simulink model "IntModelY1_2022a"  (R2022a)
settings: Solver=VariableStepAuto  StartTime=0.0  StopTime=inf  RelTol=1e-3
model workspace (MAT data in the model file):
  firstWarning = 1
  originalScenarioChecksum = '114339432DE22364D47BB28FC96DC10C'
undefined symbols (not defined in the file): Acceleration, ActorID, AngularVelocity, curvature, curvatureAhd, DefaultGear, DEND_B, DEND_S, DEND_T, direction, driving, gradbp, L, LF, LR, matlabshared, MAX_BRAKE, MAX_STEER, MAX_TORQUE, MCAR, MIN_BRAKE, MIN_STEER, MIN_TORQUE, NUMD_B, NUMD_S, NUMD_T, Pitch, Position, psi_o, R, Roll, RRdamp, SceneInfo, session, sigbuilder_block, STEER_RATIO, stopSign_ID, Tdead, thetaRefs, TL_ID, TrackWidth, Ts, ts, Vdead, Velocity, WB, X_o, xRef2s, Y_o, Yaw, yRef2s
libraries: drivingscenarioandsensors x8, drivingvehiclecontroller x2, trackingutilitieslib x2, simulink x2, robotalgslib x1, mpcadaslib x1, drivinglib x1, simulink_extras x1, autolibshared x1, vehdynlibviscommon x1, vehdynlibsteering x1
(part 3 of 3)

== stateflow chart IntModelY1_2022a/Behavioural Planner/Routing ==
  state InitialRoute
    en:
    NewRoute = 0;
  state Rerouting
    en:
    NewRoute = 1;
  (default) -> InitialRoute
  InitialRoute -> Rerouting : [ReRoute == 1]
  Rerouting -> InitialRoute : [ReRoute == 0]
  data: ReRoute input; NewRoute output

== matlab function IntModelY1_2022a/Environment & Data/Sensors & Perception/MATLAB Function1 ==
  data: EVpos input; yaw input; SceneID input; SceneInfo input; SDir output; SDist input; D2S output
function [SDir,D2S] = SceneFinder(EVpos,yaw, SceneID, SceneInfo, SDist)
D2S = zeros(10,1);
    % dist = zeros(1,length(SceneLocations));
    for j = 1:length(SceneInfo(:,1))
        distXY = SceneInfo(j,1:2) - EVpos(1:2);
        D2S(j) = norm(distXY);
        
%         if (D2S <= SDist)
%             Scene = SceneInfo(j,3); % labels {1,2,3,4} => {'TrafficLight','StopSign','RailRoadCrossing','RoundAbout'};
%             angl = atan2d(distXY(2),distXY(1));
%             angl = angl - yaw;
% %             rot = [cosd(angl) -sind(angl);sind(angl) cosd(angl)];
% %             distXY = rot*distXY';
% %             angl = atan2d(distXY(2),distXY(1));
%             
%             if angl < 0
%                 angl = angl + 360;
%             end
% 
%             if (angl > 315) || (angl <= 45) 
%                 SDir = "N";
%             elseif (angl > 225) && (angl <= 315)
%                 SDir = "E";
%             elseif (angl > 135) && (angl <= 225)
%                 SDir = "S";
%                 D2S = 1000;
%                 angl = 1000;
%                 Scene = 0;
%             elseif (angl > 45) && (angl <= 135)
%                 SDir = "W";
%             else
%                 SDir = "Error";
%             end
%             break
%         else
%             Scene = 0;
%             SDir = " ";
%             angl = 1000;
%             D2S = 1000;
%         end

    end
[val,indx] = min(D2S);

== stateflow chart IntModelY1_2022a/Behavioural Planner/Emergency Stop ==
  state EmergencyCheck
    en:
    EStop = 0;
  state Pullover
    en:
    EStop=1;
  state Stop
    en:
    EStop=2;
  Pullover -> EmergencyCheck : [TechFailure == 0]
  (default) -> EmergencyCheck
  EmergencyCheck -> Pullover [order 1] : [TechFailure == 1]
  EmergencyCheck -> Stop [order 2] : [D2O<=1]
  Stop -> EmergencyCheck : [D2O > 2]
  data: D2O input; TechFailure input; EStop output

== stateflow chart IntModelY1_2022a/Behavioural Planner/Collision Avoidance ==
  state Start
    en:
    Stuck = 0;
    ACC = 0;
    LaneChangeCmd = 0;
    %VelCmd = CurrentVelCmd;
  state Follow
    en:
    ACC = 1;
  state LaneChange
    en:
    LaneChangeCmd = 1;
  LaneChange -> Start : [LaneChanged == 1]
  (default) -> Start
  Follow -> LaneChange [order 2] : [LaneAvailable == 1 && Stuck == 1]
  Start -> Follow : [ObjAhead == 1]
  Follow -> Start [order 3] : [ObjAhead == 0]
  Follow -> Follow [order 1] : [(EgoSpeed <= MinSpeed) && after(WaitTime,sec)]{Stuck = 1;}
  data: Stuck local; ACC output; WaitTime input; ObjAhead input; MinSpeed input; LaneAvailable input; EgoSpeed input; LaneChanged input; LaneChangeCmd output

== matlab function IntModelY1_2022a/Controllers/Subsystem3/Subsystem2/MATLAB Function ==
  data: u input; accel output; decel output
function [accel, decel] = fcn(u)
if(u>0)
    accel=u; decel=0;
elseif(u<0)
    accel=0; decel=-u;
else
    accel=0;decel=0;
end

== matlab function IntModelY1_2022a/Controllers/MATLAB Function2 ==
  data: v input; RefVelCmd output; curvature input
function RefVelCmd = fcn(v,curvature)

    if abs(curvature) >= 0 && abs(curvature) <= 1e-2
        RefVelCmd = v;
    else
        r = 1/abs(curvature);
        RefVelCmd = min(v,sqrt(9.81*r*.7));
    end

== matlab function IntModelY1_2022a/Vehicle Dynamics/Info2ActorState/MATLAB Function1 ==
  data: Xdot input; Velocity output; Ydot input; Zdot input
function Velocity = fcn(Xdot, Ydot, Zdot)

Velocity = [Xdot Ydot, Zdot];

== matlab function IntModelY1_2022a/Behavioural Planner/MATLAB Function ==
  data: Dest input; D2D output; CurrentPose input
function D2D = fcn(Dest, CurrentPose)
CurrentPose(2) = -CurrentPose(2);
D2D = norm(Dest - CurrentPose(1:2)');

== matlab function IntModelY1_2022a/Vehicle Dynamics/Info2ActorState/MATLAB Function2 ==
  data: aX input; Acceleration output; aY input; aZ input
function Acceleration = fcn(aX, aY, aZ)

Acceleration = [aX aY, aZ];

== matlab function IntModelY1_2022a/Vehicle Dynamics/Info2ActorState/MATLAB Function3 ==
  data: phiDot input; AngularVelocity output; thetaDot input; psiDot input
function AngularVelocity = fcn(phiDot, thetaDot, psiDot)

AngularVelocity = [phiDot thetaDot, psiDot];

== stateflow chart IntModelY1_2022a/Vehicle Dynamics/VehicleDynamics/engine-steer-brake dynamics/GearSelection1 ==
  state Park
    CurrGear = 0;
  state Reverse
    CurrGear = -1;
  state drive
    CurrGear = 1;
  (default) -> (junction 12)
  (junction 12) -> Reverse [order 3] : [DefaultGear == -1]
  (junction 12) -> drive [order 2] : [DefaultGear == 1]
  (junction 12) -> Park [order 1] : [DefaultGear == 0]
  (junction 12) -> Park [order 4] : %fallback to park
  drive -> Park [order 2] : [gear_cmd == 0 && allowShift(vc,Tbrake)]
  Park -> Reverse [order 2] : [gear_cmd == -1 && allowShift(vc,Tbrake)]
  Park -> drive [order 1] : [gear_cmd == 1 && allowShift(vc,Tbrake)]
  Reverse -> Park [order 2] : [gear_cmd == 0 && allowShift(vc,Tbrake)]
  drive -> Reverse [order 1] : [gear_cmd == -1 && allowShift(vc,Tbrake)]
  Reverse -> drive [order 1] : [gear_cmd == 1 && allowShift(vc,Tbrake)]
  data: Tdead parameter; Vdead parameter; vel function_input; brakeT function_input; allow function_output; CurrGear output; Tbrake input; vc input; gear_cmd input; DefaultGear parameter
  function allow = allowShift(vel, brakeT):
    | function allow = allowShift(vel, brakeT)
    | allow = (abs(vel) <= Vdead) && (abs(brakeT)>Tdead);
    | end

== matlab function IntModelY1_2022a/Vehicle Dynamics/VehicleDynamics/engine-steer-brake dynamics/compute net torque ==
  data: gear input; Tnet output; Tengine input; Tbrake input; vc input
function Tnet  = net_torque(gear,Tengine,Tbrake,vc)

%  --set engine torque based on current gear selection

if (gear == 0)
    %  --vehicle is in PARK, so force engine torque to zero
    Tengine = 0;
end

Tnet = Tengine + Tbrake*tanh(5*vc);

end

== matlab function IntModelY1_2022a/Vehicle Dynamics/VehicleDynamics/engine-steer-brake dynamics/gear selection state machine ==
  data: gear output; gear_cmd input; vc input; Tbrake input; Tdead input; Vdead input
function gear = gear_change_FSM(gear_cmd,vc,Tbrake,Tdead,Vdead)

persistent GEAR

%  The vehicle gear can take on one of the following enumerated values:
%  -1 = REVERSE
%   0 = PARK
%   1 = DRIVE

%  --initialize the local persistent variables

if isempty(GEAR)
    %  --default gear at startup is PARK
    %  Note:  Change this to 1 if you want car to initialize in DRIVE
    GEAR = 0;
end


%  --evaluate the gear change finite state machine

switch GEAR
    case 0  % vehicle is in PARK
        if (gear_cmd == 1)
            %  --check to see if we can shift to DRIVE
            if ((abs(vc) <= Vdead) && (abs(Tbrake) > Tdead))
                %  --shift to DRIVE
                GEAR = 1;
            end
            
        elseif (gear_cmd == 2)
            %  --check to see if we can shift to REVERSE
            if ((abs(vc) <= Vdead) && (abs(Tbrake) > Tdead))
                %  --shift to REVERSE
                GEAR = 2;
            end
        end
        
    case 1  % vehicle is in DRIVE
        if (gear_cmd == 0)
            %  --check to see if we can shift to PARK
            if ((abs(vc) <= Vdead) && (abs(Tbrake) > Tdead))
                %  --shift to PARK
                GEAR = 0;
            end
            
        elseif (gear_cmd == 2)
            %  --check to see if we can shift to REVERSE
            if ((abs(vc) <= Vdead) && (abs(Tbrake) > Tdead))
                %  --shift to REVERSE
                GEAR = 2;
            end
        end
        
    case -1  % vehicle is in REVERSE
        if (gear_cmd == 0)
            %  --check to see if we can shift to PARK
            if ((abs(vc) <= Vdead) && (abs(Tbrake) > Tdead))
                %  --shift to PARK
                GEAR = 0;
            end
            
        elseif (gear_cmd == 1)
            %  --check to see if we can shift to DRIVE
            if ((abs(vc) <= Vdead) && (abs(Tbrake) > Tdead))
                %  --shift to DRIVE
                GEAR = 1;
            end
        end
        
    otherwise  %  --should never be here
        if (vc > Vdead)
            %  --moving forward, so must be in DRIVE
            GEAR = 1;
        elseif (vc < -Vdead)
            %  --moving backward, so must be in REVERSE
            GEAR = 2;
        else
            %  --vehicle stoppped, so must be in PARK
            GEAR = 0;
        end

end


%  --output the current actual gear setting

gear = GEAR;

return

== stateflow chart IntModelY1_2022a/Behavioural Planner/Chart ==
  settings: updateMethod=DISCRETE  sampleTime=Ts
  state Stationary
    du:
    VelCmd = 0;
    CurrentVelCmd = VelCmd;
    Navi = 0;
    Trans = 0;
    StopSim = 0;
  state Navigation
    state RailCrossing
      state Approaching
        en:
        ACC = 1;
        Tgap = 0;
        Trans = 0;
      state Stop
        en:
        VelCmd = 0;
        ACC = 0;
        CurrentVelCmd = VelCmd;
      state ExitScene
        en:
        ExitFlag = 1;
      state Transition
        en:
        Tgap = 1;
        Trans = 1;
        VelCmd = SceneSpeed;
        CurrentVelCmd = VelCmd;
      (default) -> Navigation.RailCrossing.Approaching
      Navigation.RailCrossing.Approaching -> Navigation.RailCrossing.Stop [order 1] : [D2S <= 4]
      Navigation.RailCrossing.Stop -> Navigation.RailCrossing.Transition : [RRCross == 0]
      Navigation.RailCrossing.Approaching -> Navigation.RailCrossing.ExitScene [order 2] : [SceneID ~= 10]
      Navigation.RailCrossing.Transition -> Navigation.RailCrossing.ExitScene : [SceneID == 0]
    state RoundAbout
      state Approaching
        en:
        ACC = 1;
        Trans = 0;
        Tgap = 0;
      state Stop
        en:
        VelCmd = 0;
        ACC = 0;
        CurrentVelCmd = VelCmd;
      state ExitScene
        en:
        ExitFlag = 1;
      state Transition
        en:
        Tgap = 1;
        Trans = 1;
        VelCmd = SceneSpeed;
        CurrentVelCmd = VelCmd;
      (default) -> Navigation.RoundAbout.Approaching
      Navigation.RoundAbout.Approaching -> Navigation.RoundAbout.Stop [order 1] : [D2S <= 4]
      Navigation.RoundAbout.Stop -> Navigation.RoundAbout.Transition : [Clear2Go == 1]
      Navigation.RoundAbout.Approaching -> Navigation.RoundAbout.ExitScene [order 2] : [SceneID ~= 9]
      Navigation.RoundAbout.Transition -> Navigation.RoundAbout.ExitScene : [SceneID == 0]
    state DestCheck
      en,du:
      % dest reached?
      (default) -> (junction 47)
      (junction 47) -> (junction 48) [order 1] : [D2D < 2]
      (junction 48) -> (junction 50) : {DestReached = 1;}
      (junction 47) -> (junction 49) [order 2] : {DestReached = 0;}
      (junction 50) -> (junction 49) : {StopSim = 1;}
      (junction 49) -> (junction 51)
    state TrafficLight
      state Stop
        en:
        %CurrentVelCmd = VelCmd;
        %du:
        %if D2S < 7
        % VelCmd = 0;
        %end
      state Approaching
        en:
        Tgap = 0;
        Trans = 0;
        %if TLstate(1,4) == 1
        ACC = 1;
        %else
        % ACC = 0;
        %end
      state Transition
        en:
        Trans = 1;
        ACC = 0;
        Tgap = 1;
        VelCmd = SceneSpeed;
        CurrentVelCmd = VelCmd;
      state ExitScene
        en:
        ExitFlag = 1;
      (default) -> Navigation.TrafficLight.Approaching
      Navigation.TrafficLight.Approaching -> Navigation.TrafficLight.Stop [order 1] : [D2S <= 4]
      Navigation.TrafficLight.Transition -> Navigation.TrafficLight.Approaching [order 2] : [TLstate(1,4) == 1]
      Navigation.TrafficLight.Stop -> Navigation.TrafficLight.Transition : [TLstate(1,4) == 3]
      Navigation.TrafficLight.Approaching -> Navigation.TrafficLight.Transition [order 2] : [TLstate(1,4) == 3]
      Navigation.TrafficLight.Approaching -> Navigation.TrafficLight.ExitScene [order 3] : [SceneID ~= 8]
      Navigation.TrafficLight.Transition -> Navigation.TrafficLight.ExitScene [order 1] : [SceneID == 0]
    state SceneRecognition
      en :
      VelCmd = RoadSpeed;
      CurrentVelCmd = VelCmd;
      ExitFlag = 0;
    state Go
      en:
      VelCmd = RoadSpeed;
      CurrentVelCmd = VelCmd;
      Trans = 0;
      ExitFlag = 0;
      ACC = 0;
    state StopSign
      state Approaching
        en:
        ACC = 1;
        Trans = 0;
        Tgap = 0;
      state Stop
        en:
        VelCmd = 0;
        ACC = 0;
        CurrentVelCmd = VelCmd;
      state ExitScene
        en:
        ExitFlag = 1;
      state Transition
        en:
        Trans = 1;
        ACC = 0;
        Tgap = 1;
        VelCmd = SceneSpeed;
        CurrentVelCmd = VelCmd;
      (default) -> Navigation.StopSign.Approaching
      Navigation.StopSign.Approaching -> Navigation.StopSign.Stop [order 1] : [D2S <= 7]
      Navigation.StopSign.Stop -> Navigation.StopSign.Transition : [after(3,sec) && Clear2Go == 1]
      Navigation.StopSign.Approaching -> Navigation.StopSign.ExitScene [order 2] : [SceneID ~= 7]
      Navigation.StopSign.Transition -> Navigation.StopSign.ExitScene : [SceneID == 0]
    Go -> RailCrossing [order 2] : [SceneID == 10]
    SceneRecognition -> RailCrossing [order 1] : [SceneID == 10]
    RailCrossing -> Go : [ExitFlag == 1]
    Go -> RoundAbout [order 4] : [SceneID == 9]
    SceneRecognition -> RoundAbout [order 2] : [SceneID == 9]
    RoundAbout -> Go : [ExitFlag == 1]
    (default) -> DestCheck
    SceneRecognition -> TrafficLight [order 4] : [SceneID == 8]
    DestCheck -> SceneRecognition : [DestReached == 0]
    Go -> TrafficLight [order 3] : [SceneID == 8]
    SceneRecognition -> DestCheck [order 5] : [D2D < 2]
    SceneRecognition -> StopSign [order 3] : [SceneID == 7]
    TrafficLight -> Go : [ExitFlag == 1]
    StopSign -> Go : [ExitFlag == 1]
    Go -> DestCheck [order 1] : [SceneID == 0]
    Go -> StopSign [order 5] : [SceneID == 7]
  (default) -> Stationary
  Stationary -> Navigation : [Navigate == 1]
  Navigation -> Stationary : [Navigate == 0 || DestReached == 1]
  data: TLstate input; ApproachingSpeed input; ObjectDist input; SceneSpeed input; SDist input; RRCross input; D2S input; DestReached local; Navigate input; ExitFlag local; D2D input; Clear2Go input; RoadSpeed input; CurrentVelCmd local; Navi local; VelCmd output; SceneID input; ACC output; Tgap output; Trans output; StopSim output
